simulink model "servo2019"  (R2019a)
settings: Solver=VariableStepAuto  StartTime=0.0  StopTime=10  RelTol=1e-3
values from neighbouring files (symbols this model uses):
  B = 0.1    [Servo_Param (1).m]    (also in servoParameters.m)
  Km = 1    [Servo_Param (1).m]    (also in servoParameters.m)
libraries: fl_lib x16, nesl_utility x7, ee_lib x4, fl_ps_legacy_lib x2, simulink x2
settings Model: Creator=covasanvictor  LastModifiedBy=covasanvictor
settings SolverCC: ZeroCrossAlgorithm=Adaptive
settings DataIOCC: Refine=100
settings DebuggingCC: MaskedZcDiagnostic=none  IgnoredZcDiagnostic=none

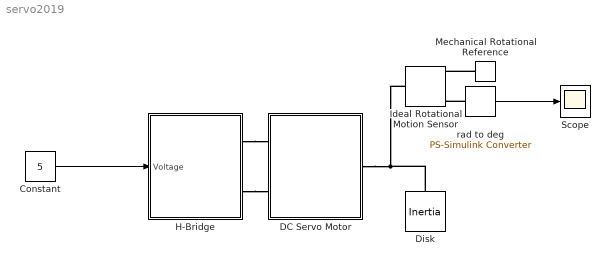
== system servo2019 ==
  Constant : Constant  Value=5
  DC Servo Motor : Subsystem
      mask Display: image('spe_servomotor_motor.jpg')
  Disk : fl_lib/Mechanical/Rotational Elements/Inertia  inertia=Jd kg*m^2  w_specify=off  w_priority=Low  w=0 rad/s  w_nominal_specify=off  w_nominal_unit=rad/s  w_nominal_value=1  t_specify=off  t_priority=None  t=0 N*m  t_nominal_specify=off  t_nominal_unit=N*m  t_nominal_value=1
  H-Bridge : Subsystem
      mask Display: image('spe_servomotor_hbridge.jpg')
  Ideal Rotational Motion Sensor : fl_lib/Mechanical/Mechanical Sensors/Ideal Rotational Motion Sensor  offset=90 deg
  Mechanical Rotational Reference : fl_lib/Mechanical/Rotational Elements/Mechanical Rotational Reference
  Scope : Scope
  rad to deg : nesl_utility/PS-Simulink Converter  PhysicalDomain=network_engine_domain  SubClassName=ps_output  LeftPortType=input  RightPortType=output  PseudoPeriodic=off  Frequencies=[]  Unit=deg  AffineConversion=off
  wires:
  Constant/1 -> H-Bridge/1(Voltage)
  rad to deg/1 -> Scope/1
  connections:
  Ideal Rotational Motion Sensor/LConn1 -- Disk/LConn1 -- DC Servo Motor/RConn1
  rad to deg/LConn1 -- Ideal Rotational Motion Sensor/RConn3
  H-Bridge/RConn2 -- DC Servo Motor/LConn2
  Mechanical Rotational Reference/LConn1 -- Ideal Rotational Motion Sensor/RConn1
  H-Bridge/RConn1 -- DC Servo Motor/LConn1

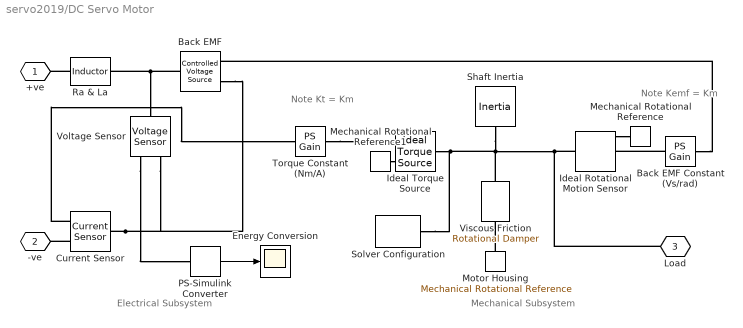
== system servo2019/DC Servo Motor ==
  note: Electrical
      | Subsystem
  note: Mechanical
      | Subsystem
  note: Note
      | Kt = Km
  note: Note
      | Kemf = Km
  Back EMF : fl_lib/Electrical/Electrical Sources/Controlled Voltage Source
  Back EMF Constant (Vs/rad) : fl_ps_legacy_lib/Legacy Physical Signals/Functions/PS Gain  gain=Km
      settings: SourceProductName=Simscape
  Current Sensor : fl_lib/Electrical/Electrical Sensors/Current Sensor
  Energy Conversion : Scope
  Ideal Rotational Motion Sensor : fl_lib/Mechanical/Mechanical Sensors/Ideal Rotational Motion Sensor  offset=90 deg
  Ideal Torque Source : fl_lib/Mechanical/Mechanical Sources/Ideal Torque Source
  Mechanical Rotational Reference : fl_lib/Mechanical/Rotational Elements/Mechanical Rotational Reference
  Mechanical Rotational Reference1 : fl_lib/Mechanical/Rotational Elements/Mechanical Rotational Reference
  Motor Housing : fl_lib/Mechanical/Rotational Elements/Mechanical Rotational Reference
  PS-Simulink Converter : nesl_utility/PS-Simulink Converter  PhysicalDomain=network_engine_domain  SubClassName=ps_output  LeftPortType=input  RightPortType=output  PseudoPeriodic=off  Frequencies=[]  Unit=1  AffineConversion=off
  Ra & La : fl_lib/Electrical/Electrical Elements/Inductor  l=La H  r=Ra Ohm  g=0 1/Ohm  i_specify=off  i_priority=None  i=0 A  i_nominal_specify=off  i_nominal_unit=A  i_nominal_value=1  v_specify=off  v_priority=None  v=0 V  v_nominal_specify=off  v_nominal_unit=V  v_nominal_value=1  i_L_specify=off  i_L_priority=High  i_L=0 A  i_L_nominal_specify=off  i_L_nominal_unit=A  i_L_nominal_value=1
  Shaft Inertia : fl_lib/Mechanical/Rotational Elements/Inertia  inertia=J kg*m^2  w_specify=off  w_priority=High  w=0 rad/s  w_nominal_specify=off  w_nominal_unit=rad/s  w_nominal_value=1  t_specify=off  t_priority=None  t=0 N*m  t_nominal_specify=off  t_nominal_unit=N*m  t_nominal_value=1
  Solver Configuration : nesl_utility/Solver Configuration  PhysicalDomain=network_engine_domain  SubClassName=solver  LeftPortType=input  RightPortType=generic  Tones=[]  Harmonics=[]  SimulateNoise=off  Profile=off  UseLocalSampling=off  EnableSwitchedLinearOptims=on  FrequencyDomain=off  UseCCode=off  RelTol=0.001  AbsTol=1e-06  MinStep=1e-09  ToWorkspace=off  RevertToSquareIcSolve=off  NumHomotopyIterations=100  PhasorMode=off  PhasorModeNumHarmonics=1  DoDC=off  ResidualTolerance=1e-9  UseLocalSolver=off  LocalSolverChoice=NE_BACKWARD_EULER_ADVANCER  LocalSolverSampleTime=.001  DoFixedCost=off  MaxNonlinIter=3  MaxModeIter=2  LinearAlgebra=Sparse  EquationFormulation=NE_TIME_EF  DelaysMemoryBudget=1024  AutomaticFiltering=on  FilteringTimeConstant=0.001  PartitionStorageMethod=AS_NEEDED  PartitionMemoryBudget=1024  PartitionMethod=FAST
  Torque Constant (Nm/A) : fl_ps_legacy_lib/Legacy Physical Signals/Functions/PS Gain  gain=Km
      settings: SourceProductName=Simscape
  Viscous Friction : fl_lib/Mechanical/Rotational Elements/Rotational Damper  D=B N*m/(rad/s)  w_specify=off  w_priority=None  w=0 rad/s  w_nominal_specify=off  w_nominal_unit=rad/s  w_nominal_value=1  t_specify=off  t_priority=None  t=0 N*m  t_nominal_specify=off  t_nominal_unit=N*m  t_nominal_value=1
  Voltage Sensor : fl_lib/Electrical/Electrical Sensors/Voltage Sensor
  +ve : PMIOPort  Tag=PMCPort  Side=Left
  -ve : PMIOPort  Tag=PMCPort  Port=2  Side=Left
  Load : PMIOPort  Port=3  Side=Right
  wires:
  PS-Simulink Converter/1 -> Energy Conversion/1
  connections:
  Ra & La/LConn1 -- +ve/RConn1
  Viscous Friction/RConn1 -- Ideal Rotational Motion Sensor/LConn1 -- Load/RConn1 -- Shaft Inertia/LConn1 -- Ideal Torque Source/LConn1 -- Solver Configuration/RConn1
  Motor Housing/LConn1 -- Viscous Friction/LConn1
  Back EMF Constant (Vs/rad)/LConn1 -- Ideal Rotational Motion Sensor/RConn2
  Ideal Rotational Motion Sensor/RConn1 -- Mechanical Rotational Reference/LConn1
  Mechanical Rotational Reference1/LConn1 -- Ideal Torque Source/RConn2
  Torque Constant (Nm/A)/RConn1 -- Ideal Torque Source/RConn1
  Back EMF/LConn1 -- Voltage Sensor/LConn1 -- Ra & La/RConn1
  Current Sensor/LConn1 -- Back EMF/RConn2 -- Voltage Sensor/RConn2
  Current Sensor/RConn2 -- -ve/RConn1
  Current Sensor/RConn1 -- Torque Constant (Nm/A)/LConn1
  Back EMF Constant (Vs/rad)/RConn1 -- Back EMF/RConn1
  Voltage Sensor/RConn1 -- PS-Simulink Converter/LConn1

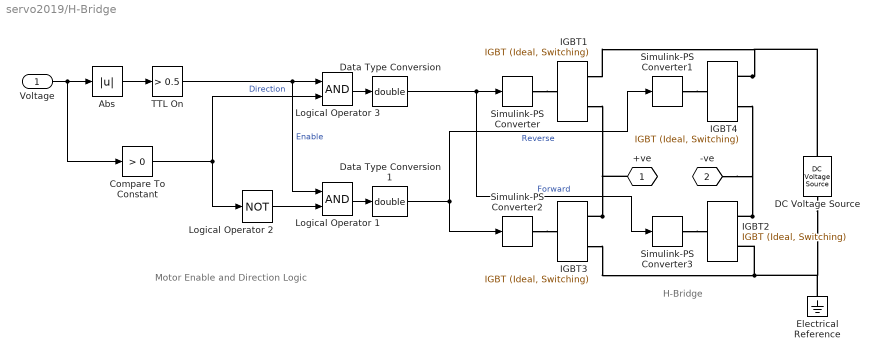
== system servo2019/H-Bridge ==
  note: Motor Enable and Direction Logic
  note: H-Bridge
  Voltage : Inport
  Abs : Abs
  Compare To Constant : simulink/Logic and Bit Operations/Compare To Constant  relop=>  const=0  OutDataTypeStr=boolean  ZeroCross=off
  DC Voltage Source : fl_lib/Electrical/Electrical Sources/DC Voltage Source  v0=6.2 V
  Data Type Conversion : DataTypeConversion  OutDataTypeStr=double
  Data Type Conversion1 : DataTypeConversion  OutDataTypeStr=double
  Electrical Reference : fl_lib/Electrical/Electrical Elements/Electrical Reference
  IGBT{1..4} (4 alike) : ee_lib/Semiconductors & Converters/IGBT (Ideal, Switching)  Vf=1 V  Ron=0.001 Ohm  Goff=1e-5 1/Ohm  Vth=0.5 V  diode_param=1  diode_Vf=0.8 V  diode_Ron=0.001 Ohm  diode_Goff=1e-5 1/Ohm  diode_C=5e-8 F  diode_iRM=-235 A  diode_iF=300 A  diode_idot=-50 A/us  diode_trr_param=1  diode_trr_factor=3  diode_trr=15 us  diode_Qrr=1.5e+3 s*uA  thermal_loss_option=2  Voff=300 V  Tau=1e-4 s  Tj=[298.15, 398.15] K  Iout_scalar=600 A  Eon_scalar=22.86e-3 J  Eoff_scalar=17.14e-3 J  Von_scalar=2.7 V  Iout_data=[0, 10, 50, 100, 200, 400, 600] A  Eon_data=[0, .29, 1.43, 2.86, 5.71, 13.14, 22.86; 0, .57, 2.63, 5.14, 10.29, 20.57, 30.29] * 1e-3 J  Eoff_data=[0, .21, 1.07, 2.14, 4.29, 9.86, 17.14; 0, .43, 1.97, 3.86, 7.71, 15.43, 22.71] * 1e-3 J  Von_data=[0, 1.1, 1.3, 1.45, 1.75, 2.25, 2.7; 0, 1, 1.15, 1.35, 1.7, 2.35, 3] V
      settings: SourceProductName=Simscape Electrical
  Logical Operator 1 : Logic  AllPortsSameDT=off  OutDataTypeStr=boolean
  Logical Operator 2 : Logic  Operator=NOT  AllPortsSameDT=off  OutDataTypeStr=boolean
  Logical Operator 3 : Logic  AllPortsSameDT=off  OutDataTypeStr=boolean
  Simulink-PS Converter{,1..3} (4 alike) : nesl_utility/Simulink-PS Converter  PhysicalDomain=network_engine_domain  SubClassName=ps_input  LeftPortType=input  RightPortType=output  PseudoPeriodic=off  Frequencies=[]  NoiseDistribution=none  NoiseParameters=[]  Unit=1  AffineConversion=off  FilteringAndDerivatives=provide  SimscapeFilterOrder=1  InputFilterTimeConstant=0.001  UdotUserProvided=0
  TTL On : simulink/Logic and Bit Operations/Compare To Constant  relop=>  const=0.5  OutDataTypeStr=boolean  ZeroCross=off
  +ve : PMIOPort  Tag=PMCPort  Side=Right
  -ve : PMIOPort  Tag=PMCPort  Port=2  Side=Right
  wires:
  Data Type Conversion1/1 -> Simulink-PS Converter1/1, Simulink-PS Converter2/1  "Reverse"
  Data Type Conversion/1 -> Simulink-PS Converter3/1, Simulink-PS Converter/1  "Forward"
  Abs/1 -> TTL On/1
  TTL On/1 -> Logical Operator 3/1, Logical Operator 1/1  "Enable"
  Voltage/1 -> Abs/1, Compare To Constant/1
  Compare To Constant/1 -> Logical Operator 3/2, Logical Operator 2/1  "Direction"
  Logical Operator 2/1 -> Logical Operator 1/2
  Logical Operator 3/1 -> Data Type Conversion/1
  Logical Operator 1/1 -> Data Type Conversion1/1
  connections:
  Simulink-PS Converter/RConn1 -- IGBT1/LConn1
  Simulink-PS Converter1/RConn1 -- IGBT4/LConn1
  Simulink-PS Converter2/RConn1 -- IGBT3/LConn1
  Simulink-PS Converter3/RConn1 -- IGBT2/LConn1
  IGBT4/RConn1 -- IGBT1/RConn1 -- DC Voltage Source/LConn1
  IGBT3/RConn1 -- IGBT1/RConn2 -- +ve/RConn1
  IGBT3/RConn2 -- IGBT2/RConn2 -- DC Voltage Source/RConn1 -- Electrical Reference/LConn1
  IGBT2/RConn1 -- IGBT4/RConn2 -- -ve/RConn1
